simulink library "hydroLib3utils_R2019B"  (R2019b)
settings: Solver=ode45  StartTime=0.0  StopTime=10.0  RelTol=1e-3
undefined symbols (not defined in the file): beta, d00, d01, d1, dP, dpn, dpn_P, dpn_T, I_Anteil_x, k_stosz, klin, omega, p0, P_Anteil_x, Qlam, Qn, Qn_P, s_dyn, s_reib, t_sw, V, V0, v_0, v_fr_min, v_min, x_max, x_min, xi
libraries: simulink x15, $bdroot x6, hydroLib3 x2
(part 1 of 2)
settings Model: Creator=bernhard  LastModifiedBy=bernh
settings DataIOCC: LimitDataPoints=on  SaveFormat=Array  ReturnWorkspaceOutputs=off
settings OptimizationCC: BlockReduction=off  BooleanDataType=off  LifeSpan=inf
settings DebuggingCC: SaveWithParameterizedLinksMsg=none  UnderspecifiedInitializationDetection=Classic  MergeDetectMultiDrivingBlocksExec=none  SignalResolutionControl=TryResolveAllWithWarning  SFUnexpectedBacktrackingDiag=warning  SFNoUnconditionalDefaultTransitionDiag=warning  SFExecutionAtInitializationDiag=none  ArithmeticOperatorsInVariantConditions=warning
settings HardwareCC: ProdBitPerPointer=32  ProdBitPerSizeT=32  ProdBitPerPtrDiffT=32  ProdLargestAtomicFloat=None  ProdIntDivRoundTo=Undefined  ProdEndianess=Unspecified  ProdWordSize=32  ProdHWDeviceType=32-bit Generic  TargetUnknown=on
settings ModelReferenceCC: PropagateSignalLabelsOutOfModel=off
settings SFSimCC: SimUseLocalCustomCode=off  CustomCodeUndefinedFunction=UseInterfaceOnly
settings RTWCC: RTWUseLocalCustomCode=off
settings CodeAppCC: StateflowObjectComments=on
settings GRTTargetCC: TargetLangStandard=C89/C90 (ANSI)
settings ConfigComp: CovMetricSettings=dw  CovSaveCumulativeToWorkspaceVar=on  CovSaveSingleToWorkspaceVar=on  CovExternalEMLEnable=off  CovSFcnEnable=off

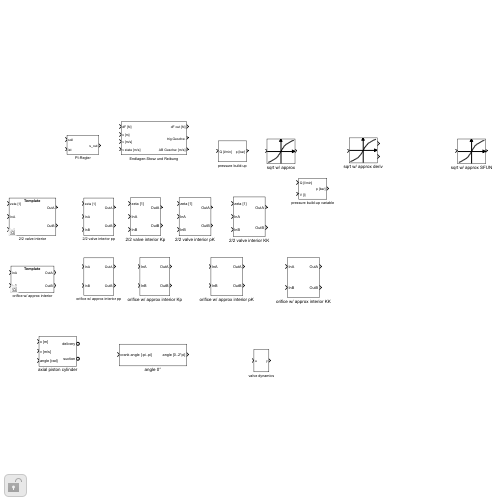
[thumbnail: Simulink's stored preview of the top-level diagram]
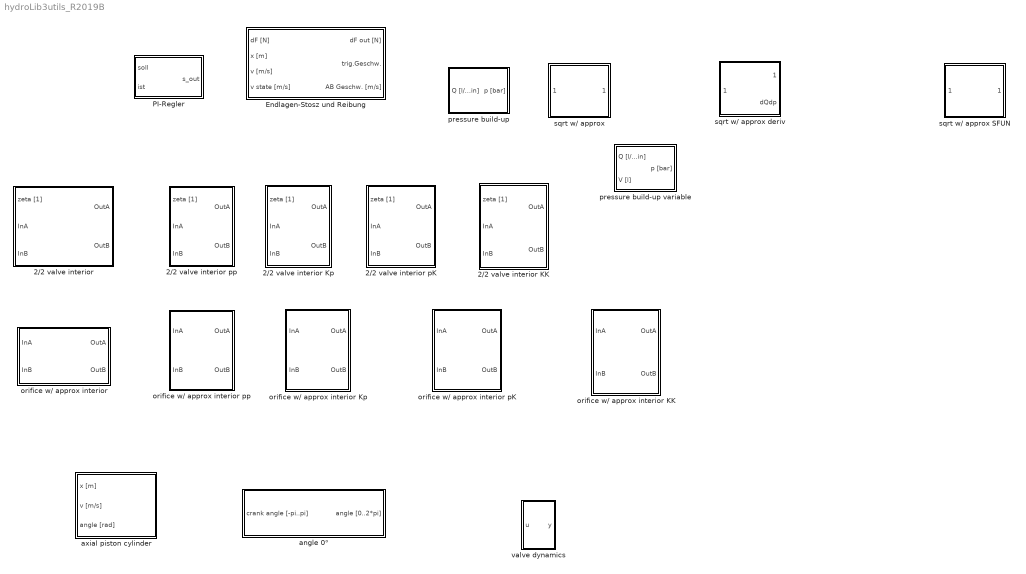
== system hydroLib3utils_R2019B ==
  2/2 valve interior : Subsystem  BlockChoice=2/2 valve interior KK
      settings: TemplateBlock=self  MemberBlocks=2/2 valve interior KK,2/2 valve interior Kp,2/2 valve interior pK,2/2 valve interior pp
  2/2 valve interior KK : Subsystem
  2/2 valve interior Kp : Subsystem
  2/2 valve interior pK : Subsystem
  2/2 valve interior pp : Subsystem
  Endlagen-Stosz und Reibung : Subsystem
  PI-Regler : Subsystem  mask{P_anteil=P_Anteil_x, I_anteil=I_Anteil_x}
      mask prompts: P_anteil "P-Anteil"; I_anteil "I-Anteil"
  angle 0° : Subsystem  mask{phi_deg=0}
      mask prompts: phi_deg "angle [°]"
      mask init:
      | phi = phi_deg*pi/180;
  axial piston cylinder : Subsystem  mask{V=dP, V0=V0, dpn=dpn_P, Qn=Qn_P, Qlam=dpn_T, phiP=3, aP=10, phiT=0, aT=0}
      mask prompts: V "stroke volume [cm³]"; V0 "dead volume [cm³]"; dpn "nominal pressure drop [bar]"; Qn "nominal flow rate [l/min]"; Qlam "lamianr flow rate [l/min]"; phiP "P-orifice angles"; aP "P-orifice values"; phiT "T-orifice angles"; aT "T-orifice values"
  orifice w/ approx interior : Subsystem  BlockChoice=orifice w/ approx interior KK
      settings: TemplateBlock=self  MemberBlocks=orifice w/ approx interior KK,orifice w/ approx interior Kp,orifice w/ approx interior pK,orifice w/ approx interior pp
  orifice w/ approx interior KK : Subsystem
  orifice w/ approx interior Kp : Subsystem
  orifice w/ approx interior pK : Subsystem
  orifice w/ approx interior pp : Subsystem
  pressure build-up : Subsystem  mask{V=V, p0=p0}
      mask prompts: V "volume [l]"; p0 "initial pressure [bar]"
      mask init:
      | K_0 = getFluidParameter('K_0');
  pressure build-up variable : Subsystem  mask{p0=p0}
      mask prompts: p0 "initial pressure [bar]"
      mask init:
      | K_0 = getFluidParameter('K_0');
  sqrt w/ approx : Subsystem  mask(Approximierte Wurzelfunktion (2. Ordn.)){Qn=Qn, dpn=dpn, Qlam=Qlam}
      mask prompts: Qn "nominal flow rate [l/min]"; dpn "nominal pressure drop [bar]"; Qlam "laminar flow rate"
      mask init:
      | pt = 2.25*dpn*(Qn/Qlam)^2;
      | 
      | kQn_dpn = Qn/sqrt(dpn);
      | 
      | a1 = Qlam/dpn;
      | a2 = 4/27*Qlam^3/(Qn^2*dpn^2);
      mask Display:
      | plot([-1.1,1.1],[0,0])
      | plot([0,0],[-1.1,1.1])
      | patch([0.9,0.9,1.1],[-0.1,0.1,0])
      | patch([-0.1,0.1,0],[0.9,0.9,1.1])
      | plot(0:0.05:0.5, 3/sqrt(2)*(0:0.05:0.5).*(1-2/3*(0:0.05:0.5)));
      | plot(0.5:0.05:1, sqrt(0.5:0.05:1));
      | plot(-0.5:0.05:0, 3/sqrt(2)*(-0.5:0.05:0).*(1+2/3*(-0.5:0.05:0)));
      | plot(-1:0.05:-0.5, -sqrt(1:-0.05:0.5));
  sqrt w/ approx SFUN : Subsystem  mask(Approximierte Wurzelfunktion (2. Ordn.)){Qn=10, dpn=1, Qlam=100}
      mask prompts: Qn "nominal flow rate [l/min]"; dpn "nominal pressure drop [bar]"; Qlam "laminar flow rate"
      mask init:
      | pt = 2.25*dpn*(Qn/Qlam)^2;
      | 
      | kQn_dpn = Qn/sqrt(dpn);
      | 
      | a1 = Qlam/dpn;
      | a2 = 4/27*Qlam^3/(Qn^2*dpn^2);
      mask Display:
      | plot([-1.1,1.1],[0,0])
      | plot([0,0],[-1.1,1.1])
      | patch([0.9,0.9,1.1],[-0.1,0.1,0])
      | patch([-0.1,0.1,0],[0.9,0.9,1.1])
      | plot(0:0.05:0.5, 3/sqrt(2)*(0:0.05:0.5).*(1-2/3*(0:0.05:0.5)));
      | plot(0.5:0.05:1, sqrt(0.5:0.05:1));
      | plot(-0.5:0.05:0, 3/sqrt(2)*(-0.5:0.05:0).*(1+2/3*(-0.5:0.05:0)));
      | plot(-1:0.05:-0.5, -sqrt(1:-0.05:0.5));
  sqrt w/ approx deriv : Subsystem  mask(Approximierte Wurzelfunktion (2. Ordn.)){Qn=Qn, dpn=dpn, Qlam=Qlam}
      mask prompts: Qn "nominal flow rate [l/min]"; dpn "nominal pressure drop [bar]"; Qlam "laminar flow rate"
      mask init:
      | pt = 2.25*dpn*(Qn/Qlam)^2;
      | 
      | kQn_dpn = Qn/sqrt(dpn);
      | 
      | a1 = Qlam/dpn;
      | a2 = 4/27*Qlam^3/(Qn^2*dpn^2);
      mask Display:
      | plot([-1.1,1.1],[0,0])
      | plot([0,0],[-1.1,1.1])
      | patch([0.9,0.9,1.1],[-0.1,0.1,0])
      | patch([-0.1,0.1,0],[0.9,0.9,1.1])
      | plot(0:0.05:0.5, 3/sqrt(2)*(0:0.05:0.5).*(1-2/3*(0:0.05:0.5)));
      | plot(0.5:0.05:1, sqrt(0.5:0.05:1));
      | plot(-0.5:0.05:0, 3/sqrt(2)*(-0.5:0.05:0).*(1+2/3*(-0.5:0.05:0)));
      | plot(-1:0.05:-0.5, -sqrt(1:-0.05:0.5));
  valve dynamics : Subsystem

== system hydroLib3utils_R2019B/2//2 valve interior ==
  zeta [1] : Inport
  InA : Inport  Port=2
  InB : Inport  Port=3
  2/2 valve interior KK : $bdroot/2//2 valve interior KK  SystemSampleTime=-1  Latency=0  AutoFrameSizeCalculation=off
  OutA : Outport
  OutB : Outport  Port=2
  wires:
  zeta [1]/1 -> 2/2 valve interior KK/1
  InA/1 -> 2/2 valve interior KK/2
  InB/1 -> 2/2 valve interior KK/3
  2/2 valve interior KK/1 -> OutA/1
  2/2 valve interior KK/2 -> OutB/1

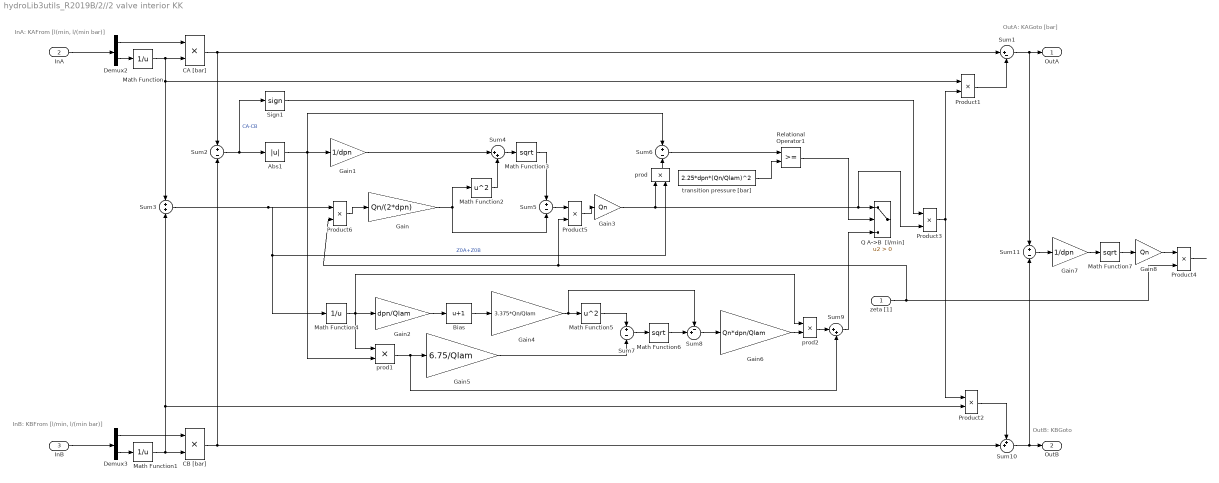
== system hydroLib3utils_R2019B/2//2 valve interior KK ==
  note: InA: KAFrom [l(min, l/(min bar)]
  note: InB: KBFrom [l/min, l/(min bar)]
  note: OutA: KAGoto [bar]
  note: OutB: KBGoto
  zeta [1] : Inport
  InA : Inport  Port=2
  InB : Inport  Port=3
  Abs1 : Abs  ZeroCross=off
  Bias : Bias  Bias=1
  CA [bar] : Product  Inputs=**  RndMeth=Zero
  CB [bar] : Product  Inputs=**  RndMeth=Zero
  Demux2 : Demux  Outputs=2
      settings: DisplayOption=none
  Demux3 : Demux  Outputs=2
      settings: DisplayOption=none
  Gain : Gain  Gain=Qn/(2*dpn)
  Gain1 : Gain  Gain=1/dpn
  Gain2 : Gain  Gain=dpn/Qlam
  Gain3 : Gain  Gain=Qn
  Gain4 : Gain  Gain=3.375*Qn/Qlam
  Gain5 : Gain  Gain=6.75/Qlam
  Gain6 : Gain  Gain=Qn*dpn/Qlam
  Gain7 : Gain  Gain=1/dpn
  Gain8 : Gain  Gain=Qn
  Math Function : Math  Operator=reciprocal  SignedPower=on  SaturateOnIntegerOverflow=on
  Math Function1 : Math  Operator=reciprocal  SignedPower=on  SaturateOnIntegerOverflow=on
  Math Function2 : Math  Operator=square  SignedPower=on  SaturateOnIntegerOverflow=on
  Math Function3 : Math  Operator=sqrt  SignedPower=on  SaturateOnIntegerOverflow=on
  Math Function4 : Math  Operator=reciprocal  SignedPower=on  SaturateOnIntegerOverflow=on
  Math Function5 : Math  Operator=square  SignedPower=on  SaturateOnIntegerOverflow=on
  Math Function6 : Math  Operator=sqrt  SignedPower=on  SaturateOnIntegerOverflow=on
  Math Function7 : Math  Operator=sqrt  SignedPower=on  SaturateOnIntegerOverflow=on
  Product{1..6} (6 alike) : Product  RndMeth=Zero
  Q A->B  [l/min] : Switch  Criteria=u2 > Threshold  ZeroCross=off
  Relational Operator1 : RelationalOperator  OutDataTypeStr=boolean  RndMeth=Nearest
  Sign1 : Signum
  Sum1 : Sum  Inputs=|+-
  Sum10 : Sum  Inputs=++|
  Sum{2,5..7,11} (5 alike) : Sum  Inputs=+|-
  Sum3 : Sum  Inputs=+|+
  Sum4 : Sum  Inputs=|++
  Sum8 : Sum  Inputs=-+|
  Sum9 : Sum  Inputs=|++
  prod : Product  Inputs=**  RndMeth=Zero
  prod1 : Product  Inputs=**  RndMeth=Zero
  prod2 : Product  Inputs=**  RndMeth=Zero
  transition pressure [bar] : Constant  Value=2.25*dpn*(Qn/Qlam)^2
  OutA : Outport
  OutB : Outport  Port=2
  wires:
  InA/1 -> Demux2/1
  Demux2/1 -> CA [bar]/1
  InB/1 -> Demux3/1
  Demux3/1 -> CB [bar]/1
  CA [bar]/1 -> Sum2/1, Sum1/1
  CB [bar]/1 -> Sum2/2, Sum10/2
  Demux2/2 -> Math Function/1
  Math Function/1 -> CA [bar]/2, Sum3/1, Product1/1
  Demux3/2 -> Math Function1/1
  Math Function1/1 -> CB [bar]/2, Sum3/2, Product2/2
  Sum3/1 -> prod/2, Math Function4/1, Product6/1  "Z0A+Z0B"
  Sum2/1 -> Abs1/1, Sign1/1  "CA-CB"
  Gain/1 -> Sum5/2, Math Function2/1
  Math Function3/1 -> Sum5/1
  prod/1 -> Sum6/2
  Sum6/1 -> Relational Operator1/1
  transition pressure [bar]/1 -> Relational Operator1/2
  Relational Operator1/1 -> Q A->B  [l/min]/2
  Gain3/1 -> prod/1, Q A->B  [l/min]/1, Product3/2
  Math Function4/1 -> Gain2/1, prod1/1, prod2/1
  Gain2/1 -> Bias/1
  Bias/1 -> Gain4/1
  Gain4/1 -> Math Function5/1, Sum8/1
  prod1/1 -> Gain5/1, Sum9/2
  Math Function5/1 -> Sum7/1
  Gain5/1 -> Sum7/2
  Sum7/1 -> Math Function6/1
  Math Function6/1 -> Sum8/2
  prod2/1 -> Sum9/1
  Gain6/1 -> prod2/2
  Sum8/1 -> Gain6/1
  Sum9/1 -> Q A->B  [l/min]/3
  Abs1/1 -> Gain1/1, Sum6/1, prod1/2
  Sign1/1 -> Product3/1
  Product3/1 -> Product1/2, Product2/1
  Product1/1 -> Sum1/2
  Sum1/1 -> OutA/1, Sum11/1
  Sum10/1 -> OutB/1, Sum11/2
  Product2/1 -> Sum10/1
  zeta [1]/1 -> Product4/2, Product5/2, Product6/2
  Math Function2/1 -> Sum4/2
  Gain1/1 -> Sum4/1
  Sum4/1 -> Math Function3/1
  Sum11/1 -> Gain7/1
  Gain7/1 -> Math Function7/1
  Math Function7/1 -> Gain8/1
  Gain8/1 -> Product4/1
  Product4/1 -> ?
  Sum5/1 -> Product5/1
  Product5/1 -> Gain3/1
  Product6/1 -> Gain/1

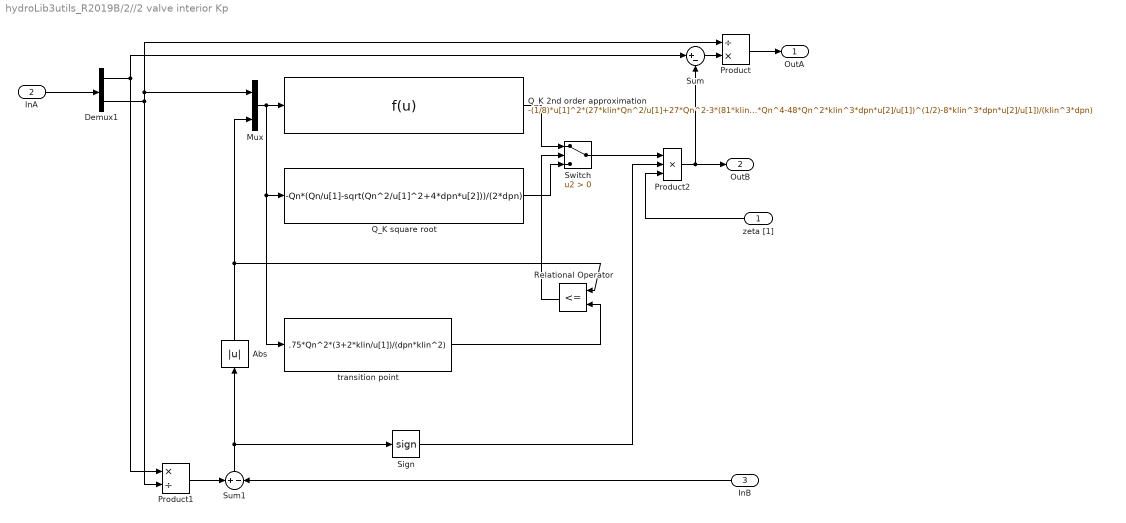
== system hydroLib3utils_R2019B/2//2 valve interior Kp ==
  zeta [1] : Inport
  InA : Inport  Port=2
  InB : Inport  Port=3
  Abs : Abs  ZeroCross=off
  Demux1 : Demux  Outputs=2
      settings: DisplayOption=none
  Mux : Mux  Inputs=2
  Product : Product  Inputs=/*  RndMeth=Zero
  Product1 : Product  Inputs=*/  RndMeth=Zero
  Product2 : Product  Inputs=3  RndMeth=Zero
  Q_K 2nd order approximation : Fcn  Expr=-(1/8)*u[1]^2*(27*klin*Qn^2/u[1]+27*Qn^2-3*(81*klin^2*Qn^4/u[1]^2+162*klin*Qn^4/u[1]+81*Qn^4-48*Qn^2*klin^3*dpn*u[2]/u[1])^(1/2)-8*klin^3*dpn*u[2]/u[1])/(klin^3*dpn)
  Q_K square root : Fcn  Expr=-Qn*(Qn/u[1]-sqrt(Qn^2/u[1]^2+4*dpn*u[2]))/(2*dpn)
  Relational Operator : RelationalOperator  Operator=<=  OutDataTypeStr=boolean  RndMeth=Nearest
  Sign : Signum
  Sum : Sum  Inputs=|+-
  Sum1 : Sum  Inputs=+|-
  Switch : Switch  Criteria=u2 > Threshold  ZeroCross=off
  transition point : Fcn  Expr=.75*Qn^2*(3+2*klin/u[1])/(dpn*klin^2)
  OutA : Outport
  OutB : Outport  Port=2
  wires:
  Switch/1 -> Product2/1
  Q_K square root/1 -> Switch/3
  Product2/1 -> Sum/2, OutB/1
  Sign/1 -> Product2/2
  Abs/1 -> Relational Operator/1, Mux/2
  Sum1/1 -> Abs/1, Sign/1
  Product/1 -> OutA/1
  Sum/1 -> Product/2
  Relational Operator/1 -> Switch/2
  transition point/1 -> Relational Operator/2
  Product1/1 -> Sum1/1
  Q_K 2nd order approximation/1 -> Switch/1
  Demux1/2 -> Mux/1, Product/1, Product1/2
  Demux1/1 -> Sum/1, Product1/1
  InA/1 -> Demux1/1
  Mux/1 -> transition point/1, Q_K square root/1, Q_K 2nd order approximation/1
  InB/1 -> Sum1/2
  zeta [1]/1 -> Product2/3

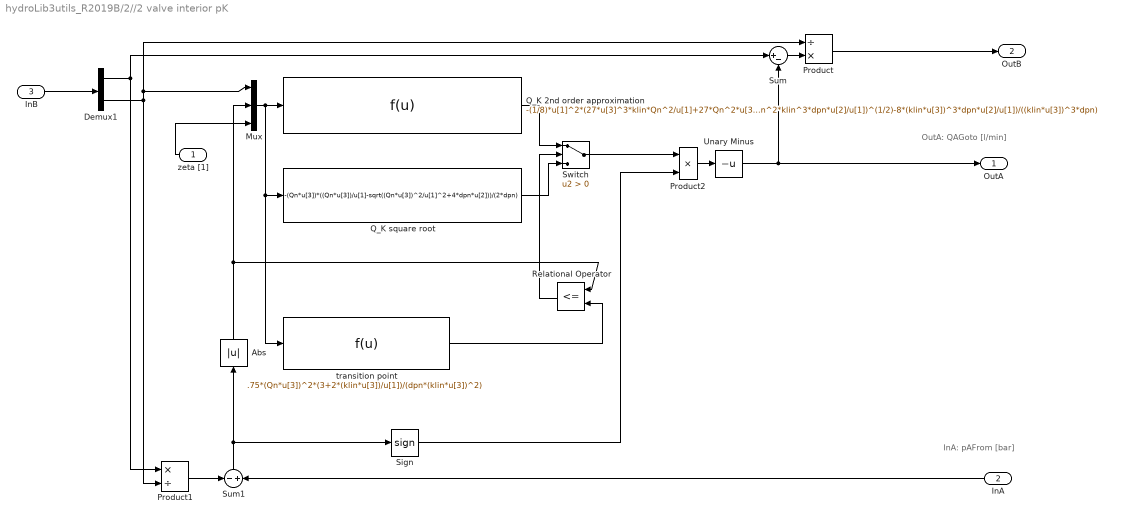
== system hydroLib3utils_R2019B/2//2 valve interior pK ==
  note: InA: pAFrom [bar]
  note: OutA: QAGoto [l/min]
  zeta [1] : Inport
  InA : Inport  Port=2
  InB : Inport  Port=3
  Abs : Abs  ZeroCross=off
  Demux1 : Demux  Outputs=2
      settings: DisplayOption=none
  Mux : Mux  Inputs=3
  Product : Product  Inputs=/*  RndMeth=Zero
  Product1 : Product  Inputs=*/  RndMeth=Zero
  Product2 : Product  RndMeth=Zero
  Q_K 2nd order approximation : Fcn  Expr=-(1/8)*u[1]^2*(27*u[3]^3*klin*Qn^2/u[1]+27*Qn^2*u[3]^2-3*(81*u[3]^6*klin^2*Qn^4/u[1]^2+162*u[3]^5*klin*Qn^4/u[1]+81*u[3]^4*Qn^4-48*u[3]^5*Qn^2*klin^3*dpn*u[2]/u[1])^(1/2)-8*(klin*u[3])^3*dpn*u[2]/u[1])/((klin*u[3])^3*dpn)
  Q_K square root : Fcn  Expr=-(Qn*u[3])*((Qn*u[3])/u[1]-sqrt((Qn*u[3])^2/u[1]^2+4*dpn*u[2]))/(2*dpn)
  Relational Operator : RelationalOperator  Operator=<=  OutDataTypeStr=boolean  RndMeth=Nearest
  Sign : Signum
  Sum : Sum  Inputs=|+-
  Sum1 : Sum  Inputs=-|+
  Switch : Switch  Criteria=u2 > Threshold  ZeroCross=off
  Unary Minus : UnaryMinus
  transition point : Fcn  Expr=.75*(Qn*u[3])^2*(3+2*(klin*u[3])/u[1])/(dpn*(klin*u[3])^2)
  OutA : Outport
  OutB : Outport  Port=2
  wires:
  InA/1 -> Sum1/2
  Mux/1 -> Q_K 2nd order approximation/1, Q_K square root/1, transition point/1
  InB/1 -> Demux1/1
  Demux1/1 -> Product1/1, Sum/1
  Demux1/2 -> Product1/2, Product/1, Mux/1
  Q_K 2nd order approximation/1 -> Switch/1
  Product1/1 -> Sum1/1
  transition point/1 -> Relational Operator/2
  Relational Operator/1 -> Switch/2
  Sum/1 -> Product/2
  Sum1/1 -> Sign/1, Abs/1
  Abs/1 -> Mux/2, Relational Operator/1
  Sign/1 -> Product2/2
  Product2/1 -> Unary Minus/1
  Q_K square root/1 -> Switch/3
  Switch/1 -> Product2/1
  Unary Minus/1 -> OutA/1, Sum/2
  Product/1 -> OutB/1
  zeta [1]/1 -> Mux/3

== system hydroLib3utils_R2019B/2//2 valve interior pp ==
  zeta [1] : Inport
  InA : Inport  Port=2
  InB : Inport  Port=3
  Product : Product  RndMeth=Zero
  Sum1 : Sum  Inputs=+|-  InputSameDT=on  SaturateOnIntegerOverflow=on  OutDataTypeStr=Inherit: Same as first input
  Unary Minus : UnaryMinus
  sqrt w/ approx : $bdroot/sqrt w// approx  Qn=Qn  dpn=dpn  Qlam=Qlam
  OutA : Outport
  OutB : Outport  Port=2
  wires:
  InB/1 -> Sum1/2
  Unary Minus/1 -> OutA/1
  InA/1 -> Sum1/1
  zeta [1]/1 -> Product/1
  Sum1/1 -> sqrt w/ approx/1
  sqrt w/ approx/1 -> Product/2
  Product/1 -> OutB/1, Unary Minus/1

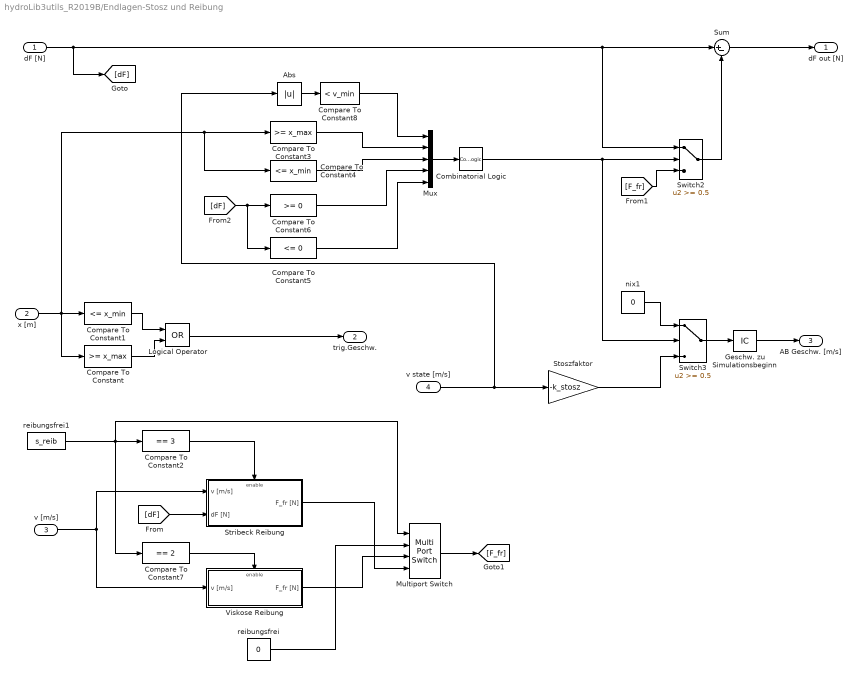
== system hydroLib3utils_R2019B/Endlagen-Stosz und Reibung ==
  dF [N] : Inport
  x [m] : Inport  Port=2
  v [m/s] : Inport  Port=3
  v state [m/s] : Inport  Port=4
  Abs : Abs
  Combinatorial Logic : CombinatorialLogic  TruthTable=[0;0;0;0; 0;0;0;0; 0;0;0;0; 0;0;0;0; 0;0;0;0; 0;1;0;0; 0;0;1;0; 0;0;0;0]
  Compare To Constant : simulink/Logic and Bit Operations/Compare To Constant  relop=>=  const=x_max  OutDataTypeStr=uint8
  Compare To Constant1 : simulink/Logic and Bit Operations/Compare To Constant  relop=<=  const=x_min  OutDataTypeStr=uint8
  Compare To Constant2 : simulink/Logic and Bit Operations/Compare To Constant  relop===  const=3  OutDataTypeStr=uint8
  Compare To Constant3 : simulink/Logic and Bit Operations/Compare To Constant  relop=>=  const=x_max  OutDataTypeStr=boolean
  Compare To Constant4 : simulink/Logic and Bit Operations/Compare To Constant  relop=<=  const=x_min  OutDataTypeStr=boolean
  Compare To Constant5 : simulink/Logic and Bit Operations/Compare To Constant  relop=<=  const=0  OutDataTypeStr=boolean
  Compare To Constant6 : simulink/Logic and Bit Operations/Compare To Constant  relop=>=  const=0  OutDataTypeStr=boolean
  Compare To Constant7 : simulink/Logic and Bit Operations/Compare To Constant  relop===  const=2  OutDataTypeStr=uint8
  Compare To Constant8 : simulink/Logic and Bit Operations/Compare To Constant  relop=<  const=v_min  OutDataTypeStr=boolean
  Geschw. zu Simulationsbeginn : InitialCondition  Value=v_0
  Logical Operator : Logic  Operator=OR  AllPortsSameDT=off  OutDataTypeStr=boolean
  Multiport Switch : MultiPortSwitch
  Mux : Mux  Inputs=5
  Stoszfaktor : Gain  Gain=-k_stosz  SaturateOnIntegerOverflow=on  OutDataTypeStr=Inherit: Same as input  ParamDataTypeStr=Inherit: Same as input
  Stribeck Reibung : Subsystem  TreatAsAtomicUnit=on
  Sum : Sum  Inputs=|+-
  Switch2 : Switch  Threshold=0.5
  Switch3 : Switch  Threshold=0.5
  Viskose Reibung : Subsystem  TreatAsAtomicUnit=on
  nix1 : Constant  Value=0
  reibungsfrei : Constant  Value=0
  reibungsfrei1 : Constant  Value=s_reib
  dF out [N] : Outport
  trig.Geschw. : Outport  Port=2
  AB Geschw. [m/s] : Outport  Port=3
  wires:
  Stribeck Reibung/1(F_fr [N]) -> Multiport Switch/4
  Viskose Reibung/1(F_fr [N]) -> Multiport Switch/3
  reibungsfrei/1 -> Multiport Switch/2
  Multiport Switch/1 -> [F_fr]
  [dF] -> Compare To Constant5/1, Compare To Constant6/1
  [F_fr] -> Switch2/3
  Compare To Constant7/1 -> Viskose Reibung/Enable
  Compare To Constant2/1 -> Stribeck Reibung/Enable
  reibungsfrei1/1 -> Multiport Switch/1, Compare To Constant7/1, Compare To Constant2/1
  v [m/s]/1 -> Viskose Reibung/1(v [m/s]), Stribeck Reibung/1(v [m/s])
  [dF] -> Stribeck Reibung/2(dF [N])
  Compare To Constant8/1 -> Mux/1
  Abs/1 -> Compare To Constant8/1
  Compare To Constant5/1 -> Mux/5
  Compare To Constant6/1 -> Mux/4
  Compare To Constant4/1 -> Mux/3
  Compare To Constant3/1 -> Mux/2
  Combinatorial Logic/1 -> Switch3/2, Switch2/2
  Mux/1 -> Combinatorial Logic/1
  Geschw. zu Simulationsbeginn/1 -> AB Geschw. [m/s]/1
  Logical Operator/1 -> trig.Geschw./1
  Compare To Constant/1 -> Logical Operator/2
  Compare To Constant1/1 -> Logical Operator/1
  x [m]/1 -> Compare To Constant/1, Compare To Constant4/1, Compare To Constant3/1, Compare To Constant1/1
  nix1/1 -> Switch3/1
  v state [m/s]/1 -> Abs/1, Stoszfaktor/1
  Switch3/1 -> Geschw. zu Simulationsbeginn/1
  Sum/1 -> dF out [N]/1
  Stoszfaktor/1 -> Switch3/3
  dF [N]/1 -> [dF], Switch2/1, Sum/1
  Switch2/1 -> Sum/2

== system hydroLib3utils_R2019B/PI-Regler ==
  soll : Inport
  ist : Inport  Port=2
  I-Anteil : Gain  Gain=I_anteil
  Integrator : Integrator  UpperSaturationLimit=0.0005  LowerSaturationLimit=-0.0005  ZeroCross=off
  P-Anteil : Gain  Gain=P_anteil
  Sum : Sum  Inputs=+-
  Sum2 : Sum  Inputs=|++
  s_out : Outport
  wires:
  soll/1 -> Sum/1
  ist/1 -> Sum/2
  Sum/1 -> I-Anteil/1, P-Anteil/1
  P-Anteil/1 -> Sum2/1
  Sum2/1 -> s_out/1
  I-Anteil/1 -> Integrator/1
  Integrator/1 -> Sum2/2

== system hydroLib3utils_R2019B/angle 0° ==
  crank angle [-pi..pi] : Inport
  Compare To Constant : simulink/Logic and Bit Operations/Compare To Constant  relop=>  const=2*pi  OutDataTypeStr=boolean  ZeroCross=off
  Compare To Constant1 : simulink/Logic and Bit Operations/Compare To Constant  relop=<  const=0  OutDataTypeStr=boolean  ZeroCross=off
  Constant : Constant  Value=phi
  Constant2 : Constant  Value=2*pi
  Ground : Ground
  Sum1 : Sum  Inputs=|++
  Sum4 : Sum  Inputs=++-
  Switch : Switch  Criteria=u2 ~= 0  ZeroCross=off
  Switch1 : Switch  Criteria=u2 ~= 0  ZeroCross=off
  angle [0..2*pi] : Outport
  wires:
  Sum4/1 -> angle [0..2*pi]/1
  Compare To Constant/1 -> Switch1/2
  crank angle [-pi..pi]/1 -> Sum1/1
  Sum1/1 -> Compare To Constant/1, Sum4/2, Compare To Constant1/1
  Constant/1 -> Sum1/2
  Switch1/1 -> Sum4/3
  Switch/1 -> Sum4/1
  Compare To Constant1/1 -> Switch/2
  Constant2/1 -> Switch/1, Switch1/1
  Ground/1 -> Switch1/3, Switch/3

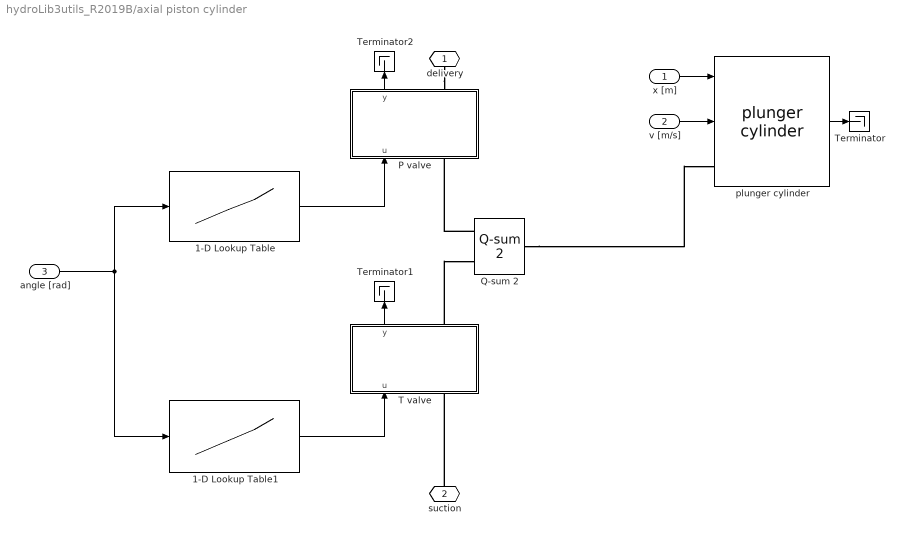
== system hydroLib3utils_R2019B/axial piston cylinder ==
  x [m] : Inport
  v [m/s] : Inport  Port=2
  angle [rad] : Inport  Port=3
  1-D Lookup Table : Lookup_n-D  NumberOfTableDimensions=1  BreakpointsForDimension1=phiP  Table=aP  RndMeth=Simplest  InputSameDT=on
  1-D Lookup Table1 : Lookup_n-D  NumberOfTableDimensions=1  BreakpointsForDimension1=phiT  Table=aT  RndMeth=Simplest  InputSameDT=on
  P valve : Subsystem  AncestorBlock=hydroLib3/valves/2//2 valve  mask{Qn=Qn, dpn=dpn, Qlam=Qlam, bcA=p, bcB=p, s_dyn=without dynamics, omega=50, xi=0.9}
      mask prompts: Qn "nominal flow rate [l/min]"; dpn "nominal pressure drop [bar]"; Qlam "laminar flow rate [l/min]"; bcA "port A boundary condition"; bcB "port B boundary condition"; s_dyn "valve dynamics"; omega "cut-off frequency [rad/s]"; xi "damping coefficient [-]"
      mask init:
      | klin =Qlam/dpn;
      | 
      | plabel = setBCs(gcb, 'AB', {'bcA', 'bcB'});
      | 
      | 
      | switch [plabel{1}(1), plabel{2}(1)]
      |     case 'pp'
      |         set_param([gcb, '/2//2 valve interior'], 'BlockChoice', '2/2 valve interior pp');
      |     case 'Kp'
      |         set_param([gcb, '/2//2 valve interior'], 'BlockChoice', '2/2 valve interior Kp');
      |     case 'pK'
      |          set_param([gcb, '/2//2 valve interior'], 'BlockChoice', '2/2 valve interior pK');
      |     case 'KK'
      |          set_param([gcb, '/2//2 valve interior'], 'BlockChoice', '2/2 valve interior KK');
      | end;
      mask TypeOptions bcA: p | K
      mask TypeOptions bcB: p | K
      mask TypeOptions s_dyn: without dynamics | PT2 behaviour
      mask Callback s_dyn:
      | maskStr = get_param(gcb,'MaskValues');
      | if  strcmp(maskStr{6}(1),'w');
      |     set_param(gcb,'MaskVisibilities',{'on';'on';'on';'on';'on';'on'; 'off';'off'});
      | else
      |     set_param(gcb,'MaskVisibilities',{'on';'on';'on';'on';'on';'on'; 'on';'on'});
      | end
      mask Display:
      | plot([0,0,1,1,0],[0,1,1,0,0]  )
      | plot([0,0,1,1,0],[0,1,1,0,0]+1)
      | plot([0,0,.5,.5,0],[0,1,1,0,0]+2)
      | plot([0,.5],[2.6,2.4])
      | 
      | plot([.25 0 .5 0 .5 0 .5 .25],[0 1 3 5 7 9 11 12]/24 -0.5)
      | 
      | plot([-1,-1]*0.1,[0,2])
      | plot([ 1, 1]*0.1+1,[0,2])
      | 
      | 
      | 
      | plot([0,1],[1.5,1.5])
      | patch(1-[0,1,1,0]*0.35, [1,1.5,0.5,1]*0.2+1.3, [0 0 0])
      | patch([0,1,1,0]*0.35,[1,1.5,0.5,1]*0.2+1.3,[0 0 0])
      | 
      | plot([0,0.2],[0.5,0.5])
      | plot([0.8,1],[0.5,0.5])
      | plot([0.2,0.2],[0.35,0.65])
      | plot([0.8,0.8],[0.35,0.65])
      | 
      | plot(0,3.5)
      | 
      | 
      | 
      | text(-0.35,0.8,plabel{1},'HorizontalAlignment','center')
      | plot([-0.1 -0.6],[0.5 0.5])
      | 
      | text(1.4,0.8,plabel{2},'HorizontalAlignment','center')
      | plot([1.1 1.6],[0.5 0.5])
      | 
      | text(-0.35,2.7,'s','HorizontalAlignment','center')
      | plot([0, -0.6],[2.5 2.5])
      | 
      | text(1.4,2.7,'y','HorizontalAlignment','center')
      | plot([0.5 1.6], [2.5 2.5])
  Q-sum 2 : hydroLib3/basic elements/Q-sum 2  SystemSampleTime=-1  Latency=0  AutoFrameSizeCalculation=off
      link override QAFrom: GotoTag=Tag1
      link override QAGoto: GotoTag=Tag2
      link override QBFrom: GotoTag=Tag3
      link override QBGoto: GotoTag=Tag4
      link override pOFrom: GotoTag=Tag5
      link override pOGoto: GotoTag=Tag6
      settings: SourceProductName=hydroLib3
  T valve : Subsystem  AncestorBlock=hydroLib3/valves/2//2 valve  mask{Qn=Qn, dpn=dpn, Qlam=Qlam, bcA=p, bcB=p, s_dyn=without dynamics, omega=50, xi=0.9}
      mask prompts: Qn "nominal flow rate [l/min]"; dpn "nominal pressure drop [bar]"; Qlam "laminar flow rate [l/min]"; bcA "port A boundary condition"; bcB "port B boundary condition"; s_dyn "valve dynamics"; omega "cut-off frequency [rad/s]"; xi "damping coefficient [-]"
      mask init: same as hydroLib3utils_R2019B/axial piston cylinder/P valve
      mask TypeOptions bcA: p | K
      mask TypeOptions bcB: p | K
      mask TypeOptions s_dyn: without dynamics | PT2 behaviour
      mask Callback s_dyn:
      | maskStr = get_param(gcb,'MaskValues');
      | if  strcmp(maskStr{6}(1),'w');
      |     set_param(gcb,'MaskVisibilities',{'on';'on';'on';'on';'on';'on'; 'off';'off'});
      | else
      |     set_param(gcb,'MaskVisibilities',{'on';'on';'on';'on';'on';'on'; 'on';'on'});
      | end
      mask Display:
      | plot([0,0,1,1,0],[0,1,1,0,0]  )
      | plot([0,0,1,1,0],[0,1,1,0,0]+1)
      | plot([0,0,.5,.5,0],[0,1,1,0,0]+2)
      | plot([0,.5],[2.6,2.4])
      | 
      | plot([.25 0 .5 0 .5 0 .5 .25],[0 1 3 5 7 9 11 12]/24 -0.5)
      | 
      | plot([-1,-1]*0.1,[0,2])
      | plot([ 1, 1]*0.1+1,[0,2])
      | 
      | 
      | 
      | plot([0,1],[1.5,1.5])
      | patch(1-[0,1,1,0]*0.35, [1,1.5,0.5,1]*0.2+1.3, [0 0 0])
      | patch([0,1,1,0]*0.35,[1,1.5,0.5,1]*0.2+1.3,[0 0 0])
      | 
      | plot([0,0.2],[0.5,0.5])
      | plot([0.8,1],[0.5,0.5])
      | plot([0.2,0.2],[0.35,0.65])
      | plot([0.8,0.8],[0.35,0.65])
      | 
      | plot(0,3.5)
      | 
      | 
      | 
      | text(-0.35,0.8,plabel{1},'HorizontalAlignment','center')
      | plot([-0.1 -0.6],[0.5 0.5])
      | 
      | text(1.4,0.8,plabel{2},'HorizontalAlignment','center')
      | plot([1.1 1.6],[0.5 0.5])
      | 
      | text(-0.35,2.7,'s','HorizontalAlignment','center')
      | plot([0, -0.6],[2.5 2.5])
      | 
      | text(1.4,2.7,'y','HorizontalAlignment','center')
      | plot([0.5 1.6], [2.5 2.5])
  Terminator : Terminator
  Terminator1 : Terminator
  Terminator2 : Terminator
  plunger cylinder : hydroLib3/cylinders/plunger cylinder  Dp=sqrt(2*V/pi)  s=100  V0=1e-3*(V0+V/2)  p0=1
      settings: SourceProductName=hydroLib3
  delivery : PMIOPort  Side=Right
  suction : PMIOPort  Port=2  Side=Right
  wires:
  plunger cylinder/1 -> Terminator/1
  v [m/s]/1 -> plunger cylinder/2
  x [m]/1 -> plunger cylinder/1
  T valve/1(y) -> Terminator1/1
  P valve/1(y) -> Terminator2/1
  angle [rad]/1 -> 1-D Lookup Table1/1, 1-D Lookup Table/1
  1-D Lookup Table/1 -> P valve/1(u)
  1-D Lookup Table1/1 -> T valve/1(u)
  connections:
  Q-sum 2/RConn1 -- plunger cylinder/LConn1
  delivery/RConn1 -- P valve/RConn1
  suction/RConn1 -- T valve/LConn1
  T valve/RConn1 -- Q-sum 2/LConn2
  Q-sum 2/LConn1 -- P valve/LConn1

== system hydroLib3utils_R2019B/orifice w// approx interior ==
  InA : Inport
  InB : Inport  Port=2
  orifice w/ approx interior KK : $bdroot/orifice w// approx interior KK  SystemSampleTime=-1  Latency=0  AutoFrameSizeCalculation=off
  OutA : Outport
  OutB : Outport  Port=2
  wires:
  InA/1 -> orifice w/ approx interior KK/1
  InB/1 -> orifice w/ approx interior KK/2
  orifice w/ approx interior KK/1 -> OutA/1
  orifice w/ approx interior KK/2 -> OutB/1

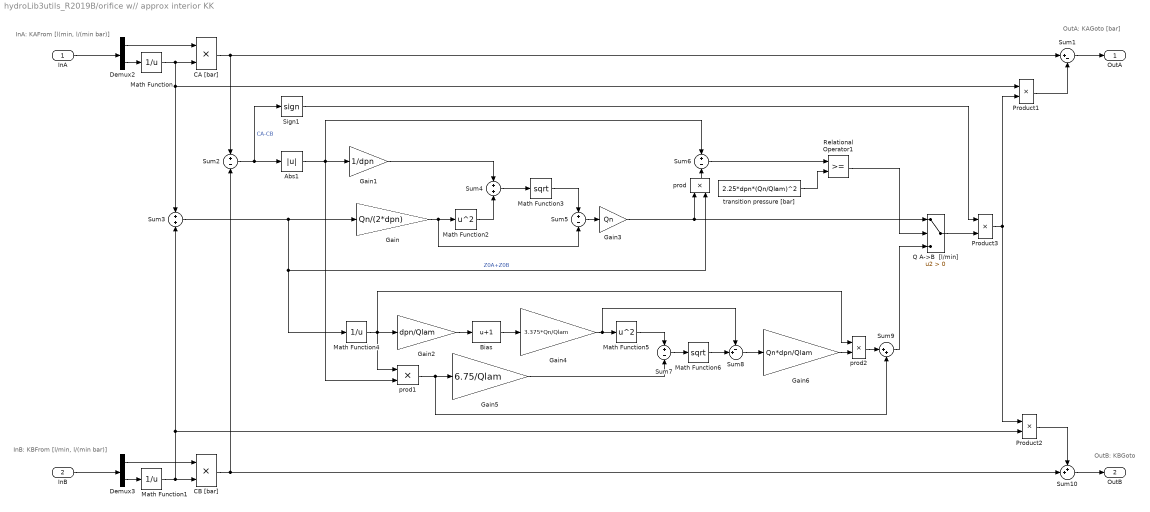
== system hydroLib3utils_R2019B/orifice w// approx interior KK ==
  note: OutB: KBGoto
  note: OutA: KAGoto [bar]
  note: InB: KBFrom [l/min, l/(min bar)]
  note: InA: KAFrom [l(min, l/(min bar)]
  InA : Inport
  InB : Inport  Port=2
  Abs1 : Abs  ZeroCross=off
  Bias : Bias  Bias=1
  CA [bar] : Product  Inputs=**  RndMeth=Zero
  CB [bar] : Product  Inputs=**  RndMeth=Zero
  Demux2 : Demux  Outputs=2
      settings: DisplayOption=none
  Demux3 : Demux  Outputs=2
      settings: DisplayOption=none
  Gain : Gain  Gain=Qn/(2*dpn)
  Gain1 : Gain  Gain=1/dpn
  Gain2 : Gain  Gain=dpn/Qlam
  Gain3 : Gain  Gain=Qn
  Gain4 : Gain  Gain=3.375*Qn/Qlam
  Gain5 : Gain  Gain=6.75/Qlam
  Gain6 : Gain  Gain=Qn*dpn/Qlam
  Math Function : Math  Operator=reciprocal  SignedPower=on  SaturateOnIntegerOverflow=on
  Math Function1 : Math  Operator=reciprocal  SignedPower=on  SaturateOnIntegerOverflow=on
  Math Function2 : Math  Operator=square  SignedPower=on  SaturateOnIntegerOverflow=on
  Math Function3 : Math  Operator=sqrt  SignedPower=on  SaturateOnIntegerOverflow=on
  Math Function4 : Math  Operator=reciprocal  SignedPower=on  SaturateOnIntegerOverflow=on
  Math Function5 : Math  Operator=square  SignedPower=on  SaturateOnIntegerOverflow=on
  Math Function6 : Math  Operator=sqrt  SignedPower=on  SaturateOnIntegerOverflow=on
  Product1 : Product  RndMeth=Zero
  Product2 : Product  RndMeth=Zero
  Product3 : Product  RndMeth=Zero
  Q A->B  [l/min] : Switch  Criteria=u2 > Threshold  ZeroCross=off
  Relational Operator1 : RelationalOperator  OutDataTypeStr=boolean  RndMeth=Nearest
  Sign1 : Signum
  Sum1 : Sum  Inputs=|+-
  Sum10 : Sum  Inputs=++|
  Sum{2,5..7} (4 alike) : Sum  Inputs=+|-
  Sum3 : Sum  Inputs=+|+
  Sum4 : Sum  Inputs=+|+
  Sum8 : Sum  Inputs=-+|
  Sum9 : Sum  Inputs=|++
  prod : Product  Inputs=**  RndMeth=Zero
  prod1 : Product  Inputs=**  RndMeth=Zero
  prod2 : Product  Inputs=**  RndMeth=Zero
  transition pressure [bar] : Constant  Value=2.25*dpn*(Qn/Qlam)^2
  OutA : Outport
  OutB : Outport  Port=2
  wires:
  Product2/1 -> Sum10/1
  Sum10/1 -> OutB/1
  Sum1/1 -> OutA/1
  Product1/1 -> Sum1/2
  Product3/1 -> Product2/1, Product1/2
  Sign1/1 -> Product3/1
  Q A->B  [l/min]/1 -> Product3/2
  Abs1/1 -> prod1/2, Sum6/1, Gain1/1
  Sum9/1 -> Q A->B  [l/min]/3
  Sum8/1 -> Gain6/1
  Gain6/1 -> prod2/2
  prod2/1 -> Sum9/1
  Math Function6/1 -> Sum8/2
  Sum7/1 -> Math Function6/1
  Gain5/1 -> Sum7/2
  Math Function5/1 -> Sum7/1
  prod1/1 -> Sum9/2, Gain5/1
  Gain4/1 -> Sum8/1, Math Function5/1
  Bias/1 -> Gain4/1
  Gain2/1 -> Bias/1
  Math Function4/1 -> prod2/1, prod1/1, Gain2/1
  Gain3/1 -> Q A->B  [l/min]/1, prod/1
  Relational Operator1/1 -> Q A->B  [l/min]/2
  transition pressure [bar]/1 -> Relational Operator1/2
  Sum6/1 -> Relational Operator1/1
  prod/1 -> Sum6/2
  Sum5/1 -> Gain3/1
  Math Function3/1 -> Sum5/1
  Sum4/1 -> Math Function3/1
  Gain1/1 -> Sum4/1
  Math Function2/1 -> Sum4/2
  Gain/1 -> Sum5/2, Math Function2/1
  Sum2/1 -> Sign1/1, Abs1/1  "CA-CB"
  Sum3/1 -> Math Function4/1, prod/2, Gain/1  "Z0A+Z0B"
  Math Function1/1 -> Product2/2, Sum3/2, CB [bar]/2
  Demux3/2 -> Math Function1/1
  Math Function/1 -> Product1/1, Sum3/1, CA [bar]/2
  Demux2/2 -> Math Function/1
  CB [bar]/1 -> Sum10/2, Sum2/2
  CA [bar]/1 -> Sum1/1, Sum2/1
  Demux3/1 -> CB [bar]/1
  InB/1 -> Demux3/1
  Demux2/1 -> CA [bar]/1
  InA/1 -> Demux2/1

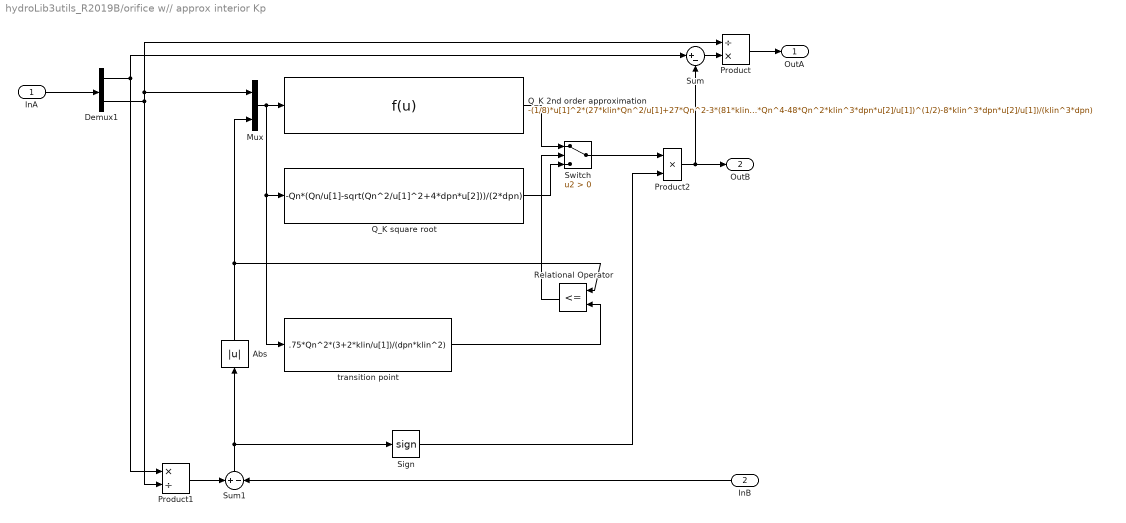
== system hydroLib3utils_R2019B/orifice w// approx interior Kp ==
  InA : Inport
  InB : Inport  Port=2
  Abs : Abs  ZeroCross=off
  Demux1 : Demux  Outputs=2
      settings: DisplayOption=none
  Mux : Mux  Inputs=2
  Product : Product  Inputs=/*  RndMeth=Zero
  Product1 : Product  Inputs=*/  RndMeth=Zero
  Product2 : Product  RndMeth=Zero
  Q_K 2nd order approximation : Fcn  Expr=-(1/8)*u[1]^2*(27*klin*Qn^2/u[1]+27*Qn^2-3*(81*klin^2*Qn^4/u[1]^2+162*klin*Qn^4/u[1]+81*Qn^4-48*Qn^2*klin^3*dpn*u[2]/u[1])^(1/2)-8*klin^3*dpn*u[2]/u[1])/(klin^3*dpn)
  Q_K square root : Fcn  Expr=-Qn*(Qn/u[1]-sqrt(Qn^2/u[1]^2+4*dpn*u[2]))/(2*dpn)
  Relational Operator : RelationalOperator  Operator=<=  OutDataTypeStr=boolean  RndMeth=Nearest
  Sign : Signum
  Sum : Sum  Inputs=|+-
  Sum1 : Sum  Inputs=+|-
  Switch : Switch  Criteria=u2 > Threshold  ZeroCross=off
  transition point : Fcn  Expr=.75*Qn^2*(3+2*klin/u[1])/(dpn*klin^2)
  OutA : Outport
  OutB : Outport  Port=2
  wires:
  InB/1 -> Sum1/2
  Mux/1 -> Q_K 2nd order approximation/1, Q_K square root/1, transition point/1
  InA/1 -> Demux1/1
  Demux1/1 -> Product1/1, Sum/1
  Demux1/2 -> Product1/2, Product/1, Mux/1
  Q_K 2nd order approximation/1 -> Switch/1
  Product1/1 -> Sum1/1
  transition point/1 -> Relational Operator/2
  Relational Operator/1 -> Switch/2
  Sum/1 -> Product/2
  Product/1 -> OutA/1
  Sum1/1 -> Sign/1, Abs/1
  Abs/1 -> Mux/2, Relational Operator/1
  Sign/1 -> Product2/2
  Product2/1 -> OutB/1, Sum/2
  Q_K square root/1 -> Switch/3
  Switch/1 -> Product2/1

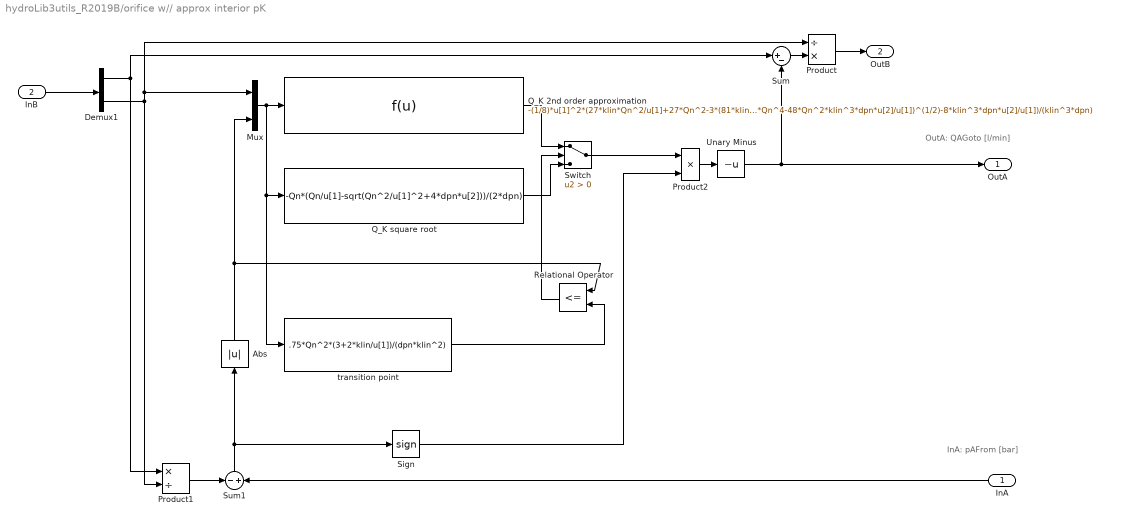
== system hydroLib3utils_R2019B/orifice w// approx interior pK ==
  note: OutA: QAGoto [l/min]
  note: InA: pAFrom [bar]
  InA : Inport
  InB : Inport  Port=2
  Abs : Abs  ZeroCross=off
  Demux1 : Demux  Outputs=2
      settings: DisplayOption=none
  Mux : Mux  Inputs=2
  Product : Product  Inputs=/*  RndMeth=Zero
  Product1 : Product  Inputs=*/  RndMeth=Zero
  Product2 : Product  RndMeth=Zero
  Q_K 2nd order approximation : Fcn  Expr=-(1/8)*u[1]^2*(27*klin*Qn^2/u[1]+27*Qn^2-3*(81*klin^2*Qn^4/u[1]^2+162*klin*Qn^4/u[1]+81*Qn^4-48*Qn^2*klin^3*dpn*u[2]/u[1])^(1/2)-8*klin^3*dpn*u[2]/u[1])/(klin^3*dpn)
  Q_K square root : Fcn  Expr=-Qn*(Qn/u[1]-sqrt(Qn^2/u[1]^2+4*dpn*u[2]))/(2*dpn)
  Relational Operator : RelationalOperator  Operator=<=  OutDataTypeStr=boolean  RndMeth=Nearest
  Sign : Signum
  Sum : Sum  Inputs=|+-
  Sum1 : Sum  Inputs=-|+
  Switch : Switch  Criteria=u2 > Threshold  ZeroCross=off
  Unary Minus : UnaryMinus
  transition point : Fcn  Expr=.75*Qn^2*(3+2*klin/u[1])/(dpn*klin^2)
  OutA : Outport
  OutB : Outport  Port=2
  wires:
  Unary Minus/1 -> Sum/2, OutA/1
  Switch/1 -> Product2/1
  Q_K square root/1 -> Switch/3
  Product2/1 -> Unary Minus/1
  Sign/1 -> Product2/2
  Abs/1 -> Relational Operator/1, Mux/2
  Sum1/1 -> Abs/1, Sign/1
  Product/1 -> OutB/1
  Sum/1 -> Product/2
  Relational Operator/1 -> Switch/2
  transition point/1 -> Relational Operator/2
  Product1/1 -> Sum1/1
  Q_K 2nd order approximation/1 -> Switch/1
  Demux1/2 -> Mux/1, Product/1, Product1/2
  Demux1/1 -> Sum/1, Product1/1
  InB/1 -> Demux1/1
  Mux/1 -> transition point/1, Q_K square root/1, Q_K 2nd order approximation/1
  InA/1 -> Sum1/2

== system hydroLib3utils_R2019B/orifice w// approx interior pp ==
  InA : Inport
  InB : Inport  Port=2
  Sum1 : Sum  Inputs=+|-  InputSameDT=on  SaturateOnIntegerOverflow=on  OutDataTypeStr=Inherit: Same as first input
  Unary Minus : UnaryMinus
  sqrt w/ approx : $bdroot/sqrt w// approx  Qn=Qn  dpn=dpn  Qlam=Qlam
  OutA : Outport
  OutB : Outport  Port=2
  wires:
  sqrt w/ approx/1 -> Unary Minus/1, OutB/1
  Sum1/1 -> sqrt w/ approx/1
  InA/1 -> Sum1/1
  Unary Minus/1 -> OutA/1
  InB/1 -> Sum1/2

== system hydroLib3utils_R2019B/pressure build-up ==
  Q [l/min] : Inport
  Gain : Gain  Gain=K_0/(V*60)
  Integrator : Integrator  InitialCondition=p0
  p [bar] : Outport
  wires:
  Integrator/1 -> p [bar]/1
  Q [l/min]/1 -> Gain/1
  Gain/1 -> Integrator/1

== system hydroLib3utils_R2019B/pressure build-up variable ==
  Q [l/min] : Inport
  V [l] : Inport  Port=2
  Divide : Product  Inputs=*/
  Gain : Gain  Gain=K_0/60
  Integrator : Integrator  InitialCondition=p0
  p [bar] : Outport
  wires:
  Q [l/min]/1 -> Gain/1
  Integrator/1 -> p [bar]/1
  Gain/1 -> Divide/1
  Divide/1 -> Integrator/1
  V [l]/1 -> Divide/2

== system hydroLib3utils_R2019B/sqrt w// approx ==
  dp [bar] : Inport
  Constant : Constant  Value=pt
  Constant1 : Constant  Value=kQn_dpn
  Constant2 : Constant  Value=a1
  Constant3 : Constant  Value=a2
  MATLAB Function : MATLAB Function  TreatAsAtomicUnit=on
  sqrt [dp] : Outport
  wires:
  MATLAB Function/1(y) -> sqrt [dp]/1
  Constant/1 -> MATLAB Function/2(pt)
  dp [bar]/1 -> MATLAB Function/1(dp)
  Constant1/1 -> MATLAB Function/3(kQn_dpn)
  Constant2/1 -> MATLAB Function/4(a1)
  Constant3/1 -> MATLAB Function/5(a2)

== system hydroLib3utils_R2019B/sqrt w// approx SFUN ==
  dp [bar] : Inport
  S-Function : S-Function  FunctionName=test_approx  Parameters=[2.25*dpn*(Qn/Qlam)^2, Qn/sqrt(dpn), Qlam/dpn, 4/27*Qlam^3/(Qn^2*dpn^2)]  SFunctionModules=test_approx_wrapper  SFunctionDeploymentMode=off  EnableBusSupport=off
  sqrt [dp] : Outport
  wires:
  dp [bar]/1 -> S-Function/1
  S-Function/1 -> sqrt [dp]/1

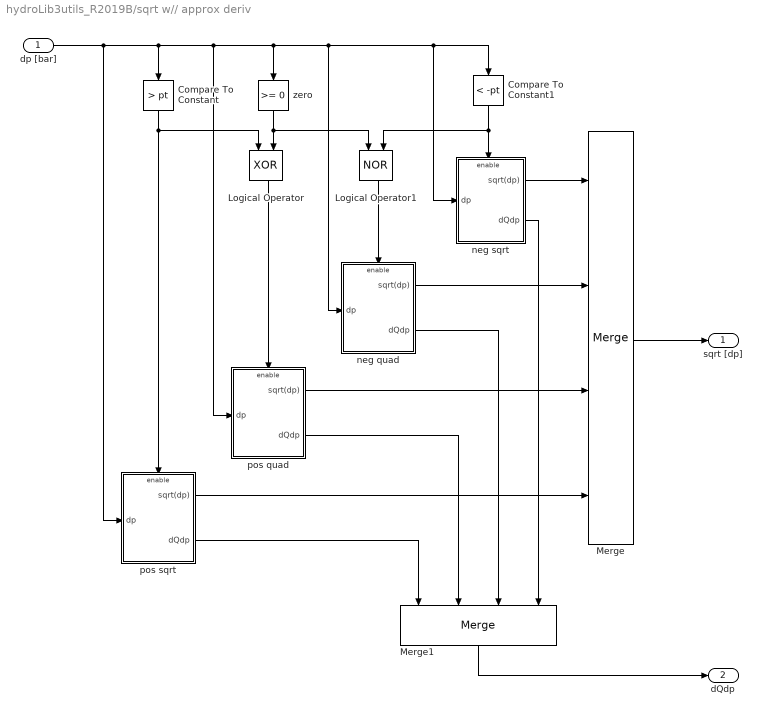
== system hydroLib3utils_R2019B/sqrt w// approx deriv ==
  dp [bar] : Inport
  Compare To Constant : simulink/Logic and Bit Operations/Compare To Constant  relop=>  const=pt  OutDataTypeStr=boolean  ZeroCross=off
  Compare To Constant1 : simulink/Logic and Bit Operations/Compare To Constant  relop=<  const=-pt  OutDataTypeStr=boolean  ZeroCross=off
  Logical Operator : Logic  Operator=XOR  AllPortsSameDT=off  OutDataTypeStr=boolean
  Logical Operator1 : Logic  Operator=NOR  OutDataTypeStr=boolean
  Merge : Merge  Inputs=4
  Merge1 : Merge  Inputs=4
  neg quad : Subsystem  TreatAsAtomicUnit=on
  neg sqrt : Subsystem  TreatAsAtomicUnit=on
  pos quad : Subsystem  TreatAsAtomicUnit=on
  pos sqrt : Subsystem  TreatAsAtomicUnit=on
  zero : simulink/Logic and Bit Operations/Compare To Zero  relop=>=  OutDataTypeStr=boolean
  sqrt [dp] : Outport
  dQdp : Outport  Port=2
  wires:
  Merge/1 -> sqrt [dp]/1
  dp [bar]/1 -> pos sqrt/1(dp), pos quad/1(dp), neg sqrt/1(dp), Compare To Constant1/1, neg quad/1(dp), zero/1, Compare To Constant/1
  pos sqrt/1(sqrt(dp)) -> Merge/4
  pos quad/1(sqrt(dp)) -> Merge/3
  neg quad/1(sqrt(dp)) -> Merge/2
  neg sqrt/1(sqrt(dp)) -> Merge/1
  Compare To Constant/1 -> pos sqrt/Enable, Logical Operator/1
  Compare To Constant1/1 -> Logical Operator1/2, neg sqrt/Enable
  Logical Operator/1 -> pos quad/Enable
  zero/1 -> Logical Operator/2, Logical Operator1/1
  Logical Operator1/1 -> neg quad/Enable
  pos sqrt/2(dQdp) -> Merge1/1
  pos quad/2(dQdp) -> Merge1/2
  neg quad/2(dQdp) -> Merge1/3
  neg sqrt/2(dQdp) -> Merge1/4
  Merge1/1 -> dQdp/1

== system hydroLib3utils_R2019B/valve dynamics ==
  u : Inport
  Constant1 : Constant  Value=s_dyn
  Merge : Merge  Inputs=3  InitialOutput=0
  PT2 : Subsystem  TreatAsAtomicUnit=on
  Saturation : Saturate  UpperLimit=1  LowerLimit=0
  Switch Case : SwitchCase  CaseConditions={1,2,3}  ShowDefaultCase=off  ZeroCross=off
  no dynamics : Subsystem  TreatAsAtomicUnit=on
  rate limiter : Subsystem  TreatAsAtomicUnit=on
  y : Outport
  wires:
  Merge/1 -> y/1
  Saturation/1 -> no dynamics/1(In1), rate limiter/1(In1), PT2/1(In1)
  PT2/1(Out1) -> Merge/3
  rate limiter/1(Out1) -> Merge/2
  no dynamics/1(Out1) -> Merge/1
  Switch Case/3 -> PT2/Action
  Switch Case/2 -> rate limiter/Action
  Switch Case/1 -> no dynamics/Action
  Constant1/1 -> Switch Case/1
  u/1 -> Saturation/1

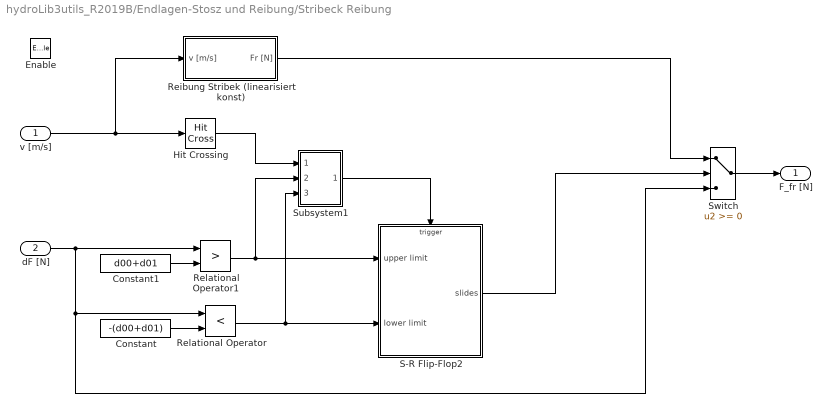
== system hydroLib3utils_R2019B/Endlagen-Stosz und Reibung/Stribeck Reibung ==
  v [m/s] : Inport
  dF [N] : Inport  Port=2
  Enable : EnablePort  PropagateVarSize=During execution
  Constant : Constant  Value=-(d00+d01)
  Constant1 : Constant  Value=d00+d01
  Hit Crossing : HitCross
  Reibung Stribek (linearisiert konst) : Subsystem
  Relational Operator : RelationalOperator  Operator=<  OutDataTypeStr=boolean  RndMeth=Nearest
  Relational Operator1 : RelationalOperator  Operator=>  OutDataTypeStr=boolean  RndMeth=Nearest
  S-R Flip-Flop2 : Subsystem  TreatAsAtomicUnit=on
  Subsystem1 : Subsystem
  Switch : Switch
  F_fr [N] : Outport
  wires:
  dF [N]/1 -> Switch/3, Relational Operator/1, Relational Operator1/1
  Switch/1 -> F_fr [N]/1
  Reibung Stribek (linearisiert konst)/1(Fr [N]) -> Switch/1
  v [m/s]/1 -> Reibung Stribek (linearisiert konst)/1(v [m/s]), Hit Crossing/1
  Subsystem1/1(Out1) -> S-R Flip-Flop2/Trigger
  Relational Operator1/1 -> Subsystem1/2(In2), S-R Flip-Flop2/1(upper limit)
  Constant1/1 -> Relational Operator1/2
  Relational Operator/1 -> Subsystem1/3(In3), S-R Flip-Flop2/2(lower limit)
  Constant/1 -> Relational Operator/2
  Hit Crossing/1 -> Subsystem1/1(In1)
  S-R Flip-Flop2/1(slides) -> Switch/2

== system hydroLib3utils_R2019B/Endlagen-Stosz und Reibung/Viskose Reibung ==
  v [m/s] : Inport
  Enable : EnablePort  PropagateVarSize=During execution
  Gain2 : Gain  Gain=d1
  F_fr [N] : Outport
  wires:
  Gain2/1 -> F_fr [N]/1
  v [m/s]/1 -> Gain2/1

== system hydroLib3utils_R2019B/axial piston cylinder/P valve ==
  u : Inport
  2/2 valve interior : Subsystem  BlockChoice=2/2 valve interior pp
      link override 2//2 valve interior pp/approx. orifice (2nd order)/Compare To Constant1/Compare: Operator=>
      link override 2//2 valve interior pp/approx. orifice (2nd order)/Compare To Constant2/Compare: Operator=<
      link override 2//2 valve interior pp/approx. orifice (2nd order)/Compare To Zero/Compare: Operator=>=
      settings: AttributesFormatString=%<BlockChoice>  TemplateBlock=hydroLib3utils/2//2 valve interior  MemberBlocks=2/2 valve interior KK,2/2 valve interior Kp,2/2 valve interior pK,2/2 valve interior pp
  pA : PMIOPort  Tag=PMCPort  Side=Left
  pB : PMIOPort  Tag=PMCPort  Port=2  Side=Right
  y : Outport
  tag scope: Tag2=global, Tag4=global
  wires:
  2/2 valve interior/2(OutB) -> [Tag4]
  [Tag1] -> 2/2 valve interior/2(InA)
  [Tag3] -> 2/2 valve interior/3(InB)
  2/2 valve interior/1(OutA) -> [Tag2]
  u/1 -> 2/2 valve interior/1(zeta [1]), y/1

== system hydroLib3utils_R2019B/axial piston cylinder/T valve ==
  u : Inport
  2/2 valve interior : Subsystem  BlockChoice=2/2 valve interior pp
      link override 2//2 valve interior pp/approx. orifice (2nd order)/Compare To Constant1/Compare: Operator=>
      link override 2//2 valve interior pp/approx. orifice (2nd order)/Compare To Constant2/Compare: Operator=<
      link override 2//2 valve interior pp/approx. orifice (2nd order)/Compare To Zero/Compare: Operator=>=
      settings: AttributesFormatString=%<BlockChoice>  TemplateBlock=hydroLib3utils/2//2 valve interior  MemberBlocks=2/2 valve interior KK,2/2 valve interior Kp,2/2 valve interior pK,2/2 valve interior pp
  pA : PMIOPort  Tag=PMCPort  Side=Left
  pB : PMIOPort  Tag=PMCPort  Port=2  Side=Right
  y : Outport
  tag scope: Tag2=global, Tag4=global
  wires:
  2/2 valve interior/2(OutB) -> [Tag4]
  u/1 -> 2/2 valve interior/1(zeta [1]), y/1
  [Tag1] -> 2/2 valve interior/2(InA)
  [Tag3] -> 2/2 valve interior/3(InB)
  2/2 valve interior/1(OutA) -> [Tag2]

== system hydroLib3utils_R2019B/sqrt w// approx deriv/neg quad ==
  dp : Inport
  Enable : EnablePort  ZeroCross=off
  Constant : Constant  Value=a1
  Gain1 : Gain  Gain=2*a2
  Gain2 : Gain  Gain=a1
  Gain3 : Gain  Gain=a2
  Math Function : Math  Operator=square  SignedPower=on  OutputSignalType=real  SaturateOnIntegerOverflow=on
  Sum : Sum  Inputs=|++
  Sum1 : Sum  Inputs=|++
  sqrt(dp) : Outport  OutputWhenDisabled=reset  InitialOutput=0
  dQdp : Outport  Port=2  OutputWhenDisabled=reset  InitialOutput=0
  wires:
  Gain3/1 -> Sum/2
  Sum/1 -> sqrt(dp)/1
  Math Function/1 -> Gain3/1
  Gain2/1 -> Sum/1
  dp/1 -> Gain2/1, Gain1/1, Math Function/1
  Constant/1 -> Sum1/1
  Gain1/1 -> Sum1/2
  Sum1/1 -> dQdp/1

== system hydroLib3utils_R2019B/sqrt w// approx deriv/neg sqrt ==
  dp : Inport
  Enable : EnablePort  ZeroCross=off
  Gain : Gain  Gain=-kQn_dpn
  Gain1 : Gain  Gain=2
  Gain2 : Gain  Gain=kQn_dpn
  Math Function : Math  Operator=reciprocal  SignedPower=on  SaturateOnIntegerOverflow=on
  Sqrt : Sqrt  SaturateOnIntegerOverflow=on
  Unary Minus : UnaryMinus
  sqrt(dp) : Outport  OutputWhenDisabled=reset  InitialOutput=0
  dQdp : Outport  Port=2  OutputWhenDisabled=reset  InitialOutput=0
  wires:
  Sqrt/1 -> Gain1/1, Gain/1
  dp/1 -> Unary Minus/1
  Unary Minus/1 -> Sqrt/1
  Gain/1 -> sqrt(dp)/1
  Gain1/1 -> Math Function/1
  Math Function/1 -> Gain2/1
  Gain2/1 -> dQdp/1

== system hydroLib3utils_R2019B/sqrt w// approx deriv/pos quad ==
  dp : Inport
  Enable : EnablePort  ZeroCross=off
  Constant : Constant  Value=a1
  Gain1 : Gain  Gain=2*a2
  Gain2 : Gain  Gain=a1
  Gain3 : Gain  Gain=a2
  Math Function : Math  Operator=square  SignedPower=on  OutputSignalType=real  SaturateOnIntegerOverflow=on
  Sum : Sum  Inputs=|+-
  Sum1 : Sum  Inputs=|+-
  sqrt(dp) : Outport  OutputWhenDisabled=reset  InitialOutput=0
  dQdp : Outport  Port=2  OutputWhenDisabled=reset  InitialOutput=0
  wires:
  dp/1 -> Gain1/1, Math Function/1, Gain2/1
  Gain2/1 -> Sum/1
  Math Function/1 -> Gain3/1
  Sum/1 -> sqrt(dp)/1
  Gain3/1 -> Sum/2
  Constant/1 -> Sum1/1
  Gain1/1 -> Sum1/2
  Sum1/1 -> dQdp/1

== system hydroLib3utils_R2019B/sqrt w// approx deriv/pos sqrt ==
  dp : Inport
  Enable : EnablePort  ZeroCross=off
  Gain : Gain  Gain=kQn_dpn
  Gain1 : Gain  Gain=2
  Gain2 : Gain  Gain=kQn_dpn
  Math Function1 : Math  Operator=reciprocal  SignedPower=on  SaturateOnIntegerOverflow=on
  Sqrt : Sqrt  SaturateOnIntegerOverflow=on
  sqrt(dp) : Outport  OutputWhenDisabled=reset  InitialOutput=0
  dQdp : Outport  Port=2  OutputWhenDisabled=reset  InitialOutput=0
  wires:
  dp/1 -> Sqrt/1
  Sqrt/1 -> Gain1/1, Gain/1
  Gain/1 -> sqrt(dp)/1
  Gain1/1 -> Math Function1/1
  Math Function1/1 -> Gain2/1
  Gain2/1 -> dQdp/1

== system hydroLib3utils_R2019B/valve dynamics/PT2 ==
  In1 : Inport
  Action Port : ActionPort
  PT2 - Ventildynamik : TransferFcn  Denominator=[1/omega^2 2*xi/omega 1]
  Out1 : Outport
  wires:
  PT2 - Ventildynamik/1 -> Out1/1
  In1/1 -> PT2 - Ventildynamik/1

== system hydroLib3utils_R2019B/valve dynamics/no dynamics ==
  In1 : Inport
  Action Port : ActionPort
  Out1 : Outport
  wires:
  In1/1 -> Out1/1

== system hydroLib3utils_R2019B/valve dynamics/rate limiter ==
  In1 : Inport
  Action Port : ActionPort
  Rate Limiter : RateLimiter  Commented=on  RisingSlewLimit=1/t_sw  FallingSlewLimit=-1/t_sw  SampleTimeMode=inherited
  Out1 : Outport
  wires:
  In1/1 -> Out1/1

== system hydroLib3utils_R2019B/Endlagen-Stosz und Reibung/Stribeck Reibung/Reibung Stribek (linearisiert konst) ==
  v [m/s] : Inport
  Abs : Abs
  Compare To Constant : simulink/Logic and Bit Operations/Compare To Constant  relop=<=  const=v_fr_min  OutDataTypeStr=boolean
  Fr_max konst : Constant  Value=(d1*v_fr_min+sign(v_fr_min)*(d00+d01*exp(-beta*abs(v_fr_min))))
  Product : Product  RndMeth=Zero
  Sign : Signum
  Subsystem2 : Subsystem
  Switch : Switch
  Fr [N] : Outport
  wires:
  Sign/1 -> Product/2
  Product/1 -> Switch/1
  Fr_max konst/1 -> Product/1
  v [m/s]/1 -> Subsystem2/1(v [m/s]), Sign/1, Abs/1
  Switch/1 -> Fr [N]/1
  Abs/1 -> Compare To Constant/1
  Compare To Constant/1 -> Switch/2
  Subsystem2/1(Fr [N]) -> Switch/3

== system hydroLib3utils_R2019B/Endlagen-Stosz und Reibung/Stribeck Reibung/S-R Flip-Flop2 ==
  upper limit : Inport
  lower limit : Inport  Port=2
  Trigger : TriggerPort  VariantControl=(inherit)
  Demux : Demux  Outputs=2
      settings: DisplayOption=none
  Logic2 : CombinatorialLogic  TruthTable=[0 0; 0 0; 0 0; 0 0; 0 1; 0 1; 1 0; 0 0; 1 0; 0 1; 1 0; 1 0; 0 0; 0 0; 0 0; 0 0]
  Logical Operator : Logic  Operator=XOR  AllPortsSameDT=off  OutDataTypeStr=boolean
  Memory : Memory  InheritSampleTime=on
  Memory1 : Memory  InheritSampleTime=on
  Mux : Mux
  Scope : Scope  NumInputPorts=2
  slides : Outport  InitialOutput=1
  wires:
  Memory/1 -> Mux/3
  Mux/1 -> Logic2/1
  Logic2/1 -> Demux/1
  Demux/2 -> Logical Operator/2, Memory1/1  "slides down"
  Demux/1 -> Scope/2, Scope/1, Logical Operator/1, Memory/1  "slides up"
  upper limit/1 -> Mux/1
  lower limit/1 -> Mux/2
  Memory1/1 -> Mux/4
  Logical Operator/1 -> slides/1

== system hydroLib3utils_R2019B/Endlagen-Stosz und Reibung/Stribeck Reibung/Subsystem1 ==
  In1 : Inport
  In2 : Inport  Port=2
  In3 : Inport  Port=3
  Detect Increase : Subsystem  AncestorBlock=|  mask(Detect Increase){vinit=0.0}
      | simulink/Logic and Bit
      | Operations/Detect
      | Increase
      mask prompts: vinit "Initial condition:"
      mask help: If the input is strictly greater than its previous value, then output TRUE, otherwise output FALSE. The initial condition determines the initial value of the previous input U/z.
      mask Display: fprintf('U > U/z')
  Detect Increase1 : Subsystem  AncestorBlock=|  mask(Detect Increase){vinit=0.0}
      | simulink/Logic and Bit
      | Operations/Detect
      | Increase
      mask prompts: vinit "Initial condition:"
      mask help: If the input is strictly greater than its previous value, then output TRUE, otherwise output FALSE. The initial condition determines the initial value of the previous input U/z.
      mask Display: fprintf('U > U/z')
  Detect Increase2 : Subsystem  AncestorBlock=|  mask(Detect Increase){vinit=0.0}
      | simulink/Logic and Bit
      | Operations/Detect
      | Increase
      mask prompts: vinit "Initial condition:"
      mask help: If the input is strictly greater than its previous value, then output TRUE, otherwise output FALSE. The initial condition determines the initial value of the previous input U/z.
      mask Display: fprintf('U > U/z')
  Logical Operator : Logic  Operator=OR  Inputs=3  AllPortsSameDT=off  OutDataTypeStr=boolean
  Out1 : Outport
  wires:
  Detect Increase2/1(Y) -> Logical Operator/3
  Detect Increase1/1(Y) -> Logical Operator/2
  Detect Increase/1(Y) -> Logical Operator/1
  In3/1 -> Detect Increase2/1(U)
  In1/1 -> Detect Increase/1(U)
  Logical Operator/1 -> Out1/1
  In2/1 -> Detect Increase1/1(U)

== system hydroLib3utils_R2019B/axial piston cylinder/P valve/2//2 valve interior ==
  zeta [1] : Inport
  InA : Inport  Port=2
  InB : Inport  Port=3
  2/2 valve interior pp : $bdroot/2//2 valve interior pp  SystemSampleTime=-1  Latency=0  AutoFrameSizeCalculation=off
  OutA : Outport
  OutB : Outport  Port=2
  wires:
  zeta [1]/1 -> 2/2 valve interior pp/1
  InA/1 -> 2/2 valve interior pp/2
  InB/1 -> 2/2 valve interior pp/3
  2/2 valve interior pp/1 -> OutA/1
  2/2 valve interior pp/2 -> OutB/1

== system hydroLib3utils_R2019B/axial piston cylinder/T valve/2//2 valve interior ==
  zeta [1] : Inport
  InA : Inport  Port=2
  InB : Inport  Port=3
  2/2 valve interior pp : $bdroot/2//2 valve interior pp  SystemSampleTime=-1  Latency=0  AutoFrameSizeCalculation=off
  OutA : Outport
  OutB : Outport  Port=2
  wires:
  zeta [1]/1 -> 2/2 valve interior pp/1
  InA/1 -> 2/2 valve interior pp/2
  InB/1 -> 2/2 valve interior pp/3
  2/2 valve interior pp/1 -> OutA/1
  2/2 valve interior pp/2 -> OutB/1

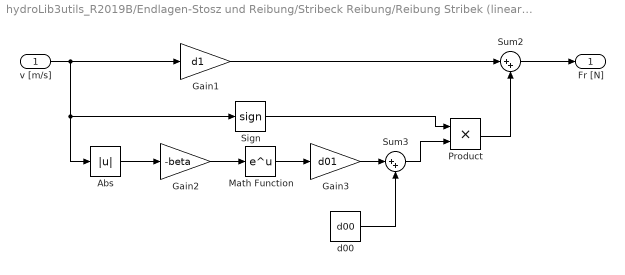
== system hydroLib3utils_R2019B/Endlagen-Stosz und Reibung/Stribeck Reibung/Reibung Stribek (linearisiert konst)/Subsystem2 ==
  v [m/s] : Inport
  Abs : Abs
  Gain1 : Gain  Gain=d1
  Gain2 : Gain  Gain=-beta
  Gain3 : Gain  Gain=d01
  Math Function : Math  SignedPower=on  SaturateOnIntegerOverflow=on
  Product : Product  RndMeth=Zero
  Sign : Signum
  Sum2 : Sum  Inputs=|++
  Sum3 : Sum  Inputs=|++
  d00 : Constant  Value=d00
  Fr [N] : Outport
  wires:
  Product/1 -> Sum2/2
  Sum3/1 -> Product/2
  Sign/1 -> Product/1
  Gain1/1 -> Sum2/1
  d00/1 -> Sum3/2
  Gain3/1 -> Sum3/1
  Math Function/1 -> Gain3/1
  Abs/1 -> Gain2/1
  Gain2/1 -> Math Function/1
  v [m/s]/1 -> Sign/1, Abs/1, Gain1/1
  Sum2/1 -> Fr [N]/1

== system hydroLib3utils_R2019B/Endlagen-Stosz und Reibung/Stribeck Reibung/Subsystem1/Detect Increase ==
  U : Inport
  FixPt Relational Operator : RelationalOperator  Operator=>  OutDataTypeStr=uint(8)  ZeroCross=off  RndMeth=Nearest
  Memory : Memory
  Y : Outport  InitialOutput=0
  wires:
  U/1 -> Memory/1, FixPt Relational Operator/1  "U(k)"
  Memory/1 -> FixPt Relational Operator/2  "U(k-1)"
  FixPt Relational Operator/1 -> Y/1  "Edge"
